simulink model "test_x_eng_nw_sim_pkt_4a_10_1"  (Simulink 7.0)
settings: Solver=ode45  StartTime=0.0  StopTime=400000  RelTol=1e-3
libraries: xbsIndex_r4 x1097, xbsReplacements_r4 x103, casper_library x28, xps_library x2, simulink x1
(part 1 of 11)
settings Model: Creator=Jason Manley  LastModifiedBy=Jason Manley
settings DebuggingCC: SaveWithParameterizedLinksMsg=none  SignalResolutionControl=TryResolveAllWithWarning  MultiTaskDSMMsg=warning  MultiTaskCondExecSysMsg=none  StrictBusMsg=None
settings RTWCC: IncludeERTFirstTime=on
settings GRTTargetCC: TargetFcnLib=ansi_tfl_tmw.mat

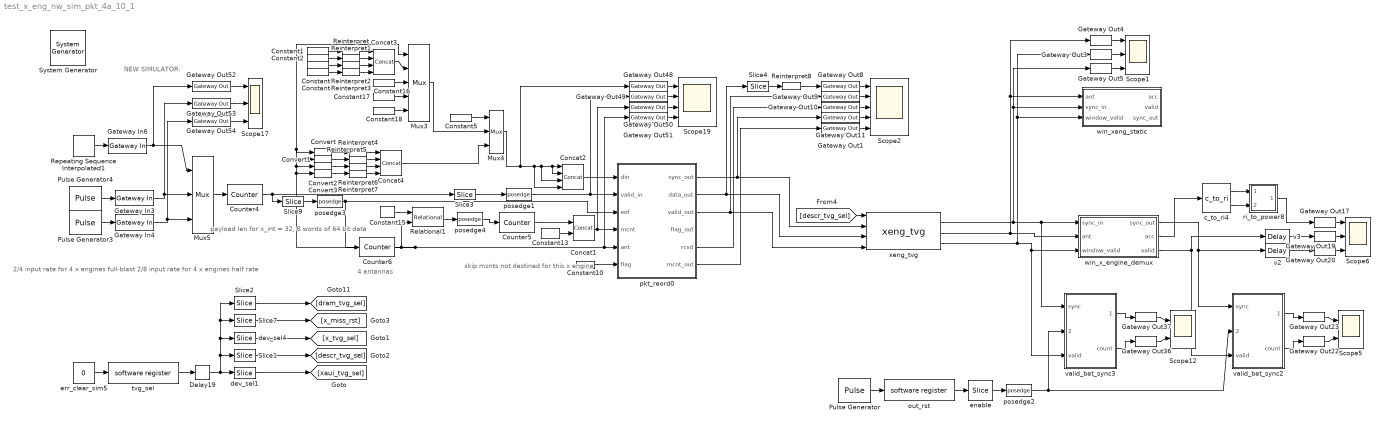
== system test_x_eng_nw_sim_pkt_4a_10_1 ==
  note: 2/4 input rate for 4 x engines full-blast
      | 2/8 input rate for 4 x engines half rate
  note: 4 antennas
  note: skip mcnts not destined
      | for this x engine
  note: payload len
      | for x_int = 32,
      | 8 words of 64 bit data
  note: NEW SIMULATOR:
  " System Generator" : xbsIndex_r4/ System Generator  Tag=genX  SystemSampleTime=-1  xilinxfamily=Virtex2  part=xc2v1000  speed=-4  package=bg575  synthesis_tool=XST  clock_wrapper=Clock Enables  directory=./netlist  testbench=off  simulink_period=1  sysclk_period=100  dcm_input_clock_period=100  incr_netlist=off  trim_vbits=Everywhere in SubSystem  dbl_ovrd=According to Block Masks  core_generation=According to Block Masks  run_coregen=off  deprecated_control=off  eval_field=0  block_type=sysgen
      settings: block_version=10.1.3
  Concat1 : xbsIndex_r4/Concat  num_inputs=2  dbl_ovrd=off  block_type=concat
      settings: block_version=10.1.3
  Concat2 : xbsIndex_r4/Concat  num_inputs=4  dbl_ovrd=off  block_type=concat
      settings: block_version=10.1.3
  Concat3 : xbsIndex_r4/Concat  num_inputs=4  dbl_ovrd=off  block_type=concat
      settings: block_version=10.1.3
  Concat4 : xbsIndex_r4/Concat  num_inputs=4  dbl_ovrd=off  block_type=concat
      settings: block_version=10.1.3
  Constant{1..4} (4 alike) : xbsIndex_r4/Constant  arith_type=Unsigned  const=0.5  n_bits=4  bin_pt=3  explicit_period=on  period=1  equ=P=C  opselect=C  inp2=PCIN>>17  opr=+  inp1=P  carry=CIN  dbl_ovrd=off  block_type=constant
  Constant10 : xbsIndex_r4/Constant  arith_type=Unsigned  const=0  n_bits=1  bin_pt=0  explicit_period=on  period=1  equ=P=C  opselect=C  inp2=PCIN>>17  opr=+  inp1=P  carry=CIN  dbl_ovrd=off  block_type=constant
  Constant13 : xbsIndex_r4/Constant  arith_type=Unsigned  const=0  n_bits=2  bin_pt=0  explicit_period=on  period=1  equ=P=C  opselect=C  inp2=PCIN>>17  opr=+  inp1=P  carry=CIN  dbl_ovrd=off  block_type=constant
  Constant15 : xbsIndex_r4/Constant  arith_type=Unsigned  const=0  n_bits=3  bin_pt=0  explicit_period=on  period=1  equ=P=C  opselect=C  inp2=PCIN>>17  opr=+  inp1=P  carry=CIN  dbl_ovrd=off  block_type=constant
  Constant16 : xbsIndex_r4/Constant  arith_type=Unsigned  const=0  n_bits=16  bin_pt=0  explicit_period=on  period=1  equ=P=C  opselect=C  inp2=PCIN>>17  opr=+  inp1=P  carry=CIN  dbl_ovrd=off  block_type=constant
  Constant17 : xbsIndex_r4/Constant  arith_type=Unsigned  const=0  n_bits=16  bin_pt=0  explicit_period=on  period=1  equ=P=C  opselect=C  inp2=PCIN>>17  opr=+  inp1=P  carry=CIN  dbl_ovrd=off  block_type=constant
  Constant18 : xbsIndex_r4/Constant  arith_type=Unsigned  const=0  n_bits=16  bin_pt=0  explicit_period=on  period=1  equ=P=C  opselect=C  inp2=PCIN>>17  opr=+  inp1=P  carry=CIN  dbl_ovrd=off  block_type=constant
  Constant5 : xbsIndex_r4/Constant  arith_type=Unsigned  const=1  n_bits=1  bin_pt=0  explicit_period=on  period=1  equ=P=C  opselect=C  inp2=PCIN>>17  opr=+  inp1=P  carry=CIN  dbl_ovrd=off  block_type=constant
  Convert{,1..3} (4 alike) : xbsIndex_r4/Convert  arith_type="Signed  (2's comp)"  n_bits=4  bin_pt=1  quantization=Truncate  overflow=Saturate  latency=0  dbl_ovrd=off  pipeline=off  block_type=convert
      settings: block_version=10.1.3
  Counter4 : xbsIndex_r4/Counter  cnt_type=Free Running  cnt_to=32  operation=Up  start_count=0  cnt_by_val=1  arith_type=Unsigned  n_bits=32  bin_pt=0  load_pin=off  rst=off  en=on  explicit_period=off  period=1  dbl_ovrd=off  use_behavioral_HDL=off  use_rpm=on  implementation=Fabric  block_type=counter
      settings: xl_area=[0, 0, 0, 0, 0, 0, 0]
  Counter5 : xbsIndex_r4/Counter  cnt_type=Free Running  cnt_to=Inf  operation=Up  start_count=0  cnt_by_val=1  arith_type=Unsigned  n_bits=48-2  bin_pt=0  load_pin=off  rst=off  en=on  explicit_period=off  period=1  dbl_ovrd=off  use_behavioral_HDL=off  use_rpm=on  implementation=Fabric  block_type=counter
      settings: xl_area=[0, 0, 0, 0, 0, 0, 0]
  Counter6 : xbsIndex_r4/Counter  cnt_type=Free Running  cnt_to=Inf  operation=Up  start_count=0  cnt_by_val=1  arith_type=Unsigned  n_bits=2  bin_pt=0  load_pin=off  rst=off  en=on  explicit_period=off  period=1  dbl_ovrd=off  use_behavioral_HDL=off  use_rpm=on  implementation=Fabric  block_type=counter
      settings: xl_area=[0, 0, 0, 0, 0, 0, 0]
  Delay19 : xbsIndex_r4/Delay  en=off  latency=2  dbl_ovrd=off  reg_retiming=off  block_type=delay
      settings: xl_area=[0, 0, 0, 0, 0, 0, 0]
  Gateway In3 : xbsIndex_r4/Gateway In  arith_type=Boolean  n_bits=8  bin_pt=6  quantization=Truncate  overflow=Wrap  period=1  dbl_ovrd=off  timing_constraint=None  locs_specified=off  LOCs={}  block_type=gatewayin
      settings: infoedit="Gateway in block.  Converts inputs of type Simulink integer, double and fixed point to  Xilinx fixed point type.<P><P>Hardware notes:  In hardware these blocks become top level input ports."  xl_area=[0, 0, 0, 0, 0, 0, 0]  block_version=10.1.3
  Gateway In4 : xbsIndex_r4/Gateway In  arith_type=Boolean  n_bits=8  bin_pt=6  quantization=Truncate  overflow=Wrap  period=1  dbl_ovrd=off  timing_constraint=None  locs_specified=off  LOCs={}  block_type=gatewayin
      settings: infoedit="Gateway in block.  Converts inputs of type Simulink integer, double and fixed point to  Xilinx fixed point type.<P><P>Hardware notes:  In hardware these blocks become top level input ports."  xl_area=[0, 0, 0, 0, 0, 0, 0]  block_version=10.1.3
  Gateway In6 : xbsIndex_r4/Gateway In  arith_type=Unsigned  n_bits=1  bin_pt=0  quantization=Truncate  overflow=Wrap  period=1  dbl_ovrd=off  timing_constraint=None  locs_specified=off  LOCs={}  block_type=gatewayin
      settings: infoedit="Gateway in block.  Converts inputs of type Simulink integer, double and fixed point to  Xilinx fixed point type.<P><P>Hardware notes:  In hardware these blocks become top level input ports."  xl_area=[0, 0, 0, 0, 0, 0, 0]  block_version=10.1.3
  Gateway Out{1,8..11,48..54} (12 alike) : xbsIndex_r4/Gateway Out  hdl_port=on  timing_constraint=None  locs_specified=off  LOCs={}  block_type=gatewayout
      settings: infoedit="Gateway out block.  Converts Xilinx fixed point inputs into ouputs of type Simulink integer, double, or fixed point.<P><P>Hardware notes:  In hardware these blocks become top level output ports or are discarded, depending on how they are configured."  xl_area=[0, 0, 0, 0, 0, 0, 0]  block_version=10.1.3
  Gateway Out{3..5,17,19..20,22..23,36..37} (10 alike) : xbsIndex_r4/Gateway Out  hdl_port=off  timing_constraint=None  locs_specified=off  LOCs={}  block_type=gatewayout
      settings: infoedit="Gateway out block.  Converts Xilinx fixed point inputs into ouputs of type Simulink integer, double, or fixed point.<P><P>Hardware notes:  In hardware these blocks become top level output ports or are discarded, depending on how they are configured."  xl_area=[0, 0, 0, 0, 0, 0, 0]  block_version=10.1.3
  Mux3 : xbsIndex_r4/Mux  inputs=4  en=off  latency=0  precision=Full  arith_type="Signed  (2's comp)"  n_bits=8  bin_pt=2  quantization=Truncate  overflow=Wrap  dbl_ovrd=off  block_type=mux
      settings: xl_area=[0, 0, 0, 0, 0, 0, 0]
  Mux4 : xbsIndex_r4/Mux  inputs=2  en=off  latency=0  precision=Full  arith_type="Signed  (2's comp)"  n_bits=8  bin_pt=2  quantization=Truncate  overflow=Wrap  dbl_ovrd=off  block_type=mux
      settings: xl_area=[0, 0, 0, 0, 0, 0, 0]
  Mux5 : xbsIndex_r4/Mux  inputs=2  en=off  latency=0  precision=Full  arith_type="Signed  (2's comp)"  n_bits=8  bin_pt=2  quantization=Truncate  overflow=Wrap  dbl_ovrd=off  block_type=mux
      settings: xl_area=[0, 0, 0, 0, 0, 0, 0]
  Pulse Generator : DiscretePulseGenerator  Period=2^15  PhaseDelay=2^14
  Pulse Generator3 : DiscretePulseGenerator  Period=4  PulseWidth=2
  Pulse Generator4 : DiscretePulseGenerator  PulseWidth=2
  Reinterpret{,1..7} (8 alike) : xbsIndex_r4/Reinterpret  force_arith_type=on  arith_type=Unsigned  force_bin_pt=on  bin_pt=0  block_type=reinterpret
      settings: infoedit="Changes signal type without altering the binary representation.   You can changed the signal between signed and unsigned, and relocate the binary point.<P><P>Hardware notes: In hardware this block costs nothing.<P><P>Example:  Suppose the input is 6 bits wide, signed, with 2 fractional bits, and the output is forced to unsigned with 0 fractional bits.  Then an input of -2.0 (1110.00 in binary 2's complement) becomes an output of 56 (111000 in binary)."  block_version=10.1.3
  Reinterpret8 : xbsIndex_r4/Reinterpret  force_arith_type=on  arith_type="Signed  (2's comp)"  force_bin_pt=on  bin_pt=3  block_type=reinterpret
      settings: infoedit="Changes signal type without altering the binary representation.   You can changed the signal between signed and unsigned, and relocate the binary point.<P><P>Hardware notes: In hardware this block costs nothing.<P><P>Example:  Suppose the input is 6 bits wide, signed, with 2 fractional bits, and the output is forced to unsigned with 0 fractional bits.  Then an input of -2.0 (1110.00 in binary 2's complement) becomes an output of 56 (111000 in binary)."  block_version=10.1.3
  Relational1 : xbsIndex_r4/Relational  mode=a=b  en=off  latency=1  dbl_ovrd=off  block_type=relational
      settings: xl_area=[0, 0, 0, 0, 0, 0, 0]  block_version=10.1.3
  Repeating Sequence Interpolated1 : simulink/Sources/Repeating Sequence Interpolated  SystemSampleTime=-1  OutValues=[0 1].'  TimeValues=[100000 300000].'  LookUpMeth=Use Input Above  tsamp=1  OutMin=[]  OutMax=[]  OutDataTypeStr=float('double')  OutputDataTypeScalingMode=Specify via dialog  OutDataType=float('double')  OutScaling=2^-10
  Scope1 : Scope  NumInputPorts=3
      settings: YMin=0~-1~0.95  YMax=1~1~1.05  SaveName=ScopeData5
  Scope12 : Scope  NumInputPorts=2
      settings: YMin=31128.7~9840  YMax=34405.3~10060  SaveName=data_into_xeng
  Scope17 : Scope  NumInputPorts=3
      settings: YMin=-1~0~0  YMax=1~1~1  SaveName=ScopeData9
  Scope19 : Scope  NumInputPorts=4
      settings: YMin=0~0~28~0  YMax=1~1~40~3  SaveName=ScopeData14
  Scope2 : Scope  NumInputPorts=5
      settings: YMin=0~0.95~0.95~-1~790  YMax=0.75~1.05~1.05~1~885
  Scope5 : Scope  NumInputPorts=2
      settings: YMin=2432~1140  YMax=2688~1150  SaveName=data_into_xeng2
  Scope6 : Scope  NumInputPorts=3
      settings: YMin=0~0~-1  YMax=1300~1~1  SaveName=ScopeData2
  Slice1 : xbsIndex_r4/Slice  nbits=2  boolean_output=off  mode=Lower Bit Location + Width  bit1=0  base1=MSB of Input  bit0=1  base0=LSB of Input  dbl_ovrd=off  block_type=slice
      settings: infoedit="Extracts a given range of bits from each input sample and presents it at the output.  The output type is ordinarily unsigned with binary point at zero, but can be Boolean when the slice is one bit wide.<P><P>Hardware notes: In hardware this block costs nothing."  block_version=10.1.3
  Slice2 : xbsIndex_r4/Slice  nbits=5  boolean_output=off  mode=Lower Bit Location + Width  bit1=0  base1=MSB of Input  bit0=9  base0=LSB of Input  dbl_ovrd=off  block_type=slice
      settings: infoedit="Extracts a given range of bits from each input sample and presents it at the output.  The output type is ordinarily unsigned with binary point at zero, but can be Boolean when the slice is one bit wide.<P><P>Hardware notes: In hardware this block costs nothing."  block_version=10.1.3
  Slice3 : xbsIndex_r4/Slice  nbits=1  boolean_output=on  mode=Lower Bit Location + Width  bit1=0  base1=MSB of Input  bit0=0  base0=LSB of Input  dbl_ovrd=off  block_type=slice
      settings: infoedit="Extracts a given range of bits from each input sample and presents it at the output.  The output type is ordinarily unsigned with binary point at zero, but can be Boolean when the slice is one bit wide.<P><P>Hardware notes: In hardware this block costs nothing."  block_version=10.1.3
  Slice4 : xbsIndex_r4/Slice  nbits=4  boolean_output=off  mode=Lower Bit Location + Width  bit1=0  base1=MSB of Input  bit0=0  base0=LSB of Input  dbl_ovrd=off  block_type=slice
      settings: infoedit="Extracts a given range of bits from each input sample and presents it at the output.  The output type is ordinarily unsigned with binary point at zero, but can be Boolean when the slice is one bit wide.<P><P>Hardware notes: In hardware this block costs nothing."  block_version=10.1.3
  Slice7 : xbsIndex_r4/Slice  nbits=1  boolean_output=on  mode=Lower Bit Location + Width  bit1=0  base1=MSB of Input  bit0=8  base0=LSB of Input  dbl_ovrd=off  block_type=slice
      settings: infoedit="Extracts a given range of bits from each input sample and presents it at the output.  The output type is ordinarily unsigned with binary point at zero, but can be Boolean when the slice is one bit wide.<P><P>Hardware notes: In hardware this block costs nothing."  block_version=10.1.3
  Slice9 : xbsIndex_r4/Slice  nbits=1  boolean_output=on  mode=Lower Bit Location + Width  bit1=0  base1=MSB of Input  bit0=4  base0=LSB of Input  dbl_ovrd=off  block_type=slice
      settings: infoedit="Extracts a given range of bits from each input sample and presents it at the output.  The output type is ordinarily unsigned with binary point at zero, but can be Boolean when the slice is one bit wide.<P><P>Hardware notes: In hardware this block costs nothing."  block_version=10.1.3
  c_to_ri4 : casper_library/Misc/c_to_ri  SystemSampleTime=-1  n_bits=16  bin_pt=6
      settings: AttributesFormatString=16_6 r/i
  dev_sel1 : xbsIndex_r4/Slice  nbits=1  boolean_output=off  mode=Lower Bit Location + Width  bit1=0  base1=MSB of Input  bit0=0  base0=LSB of Input  dbl_ovrd=off  block_type=slice
      settings: infoedit="Extracts a given range of bits from each input sample and presents it at the output.  The output type is ordinarily unsigned with binary point at zero, but can be Boolean when the slice is one bit wide.<P><P>Hardware notes: In hardware this block costs nothing."  block_version=10.1.3
  dev_sel4 : xbsIndex_r4/Slice  nbits=2  boolean_output=off  mode=Lower Bit Location + Width  bit1=0  base1=MSB of Input  bit0=3  base0=LSB of Input  dbl_ovrd=off  block_type=slice
      settings: infoedit="Extracts a given range of bits from each input sample and presents it at the output.  The output type is ordinarily unsigned with binary point at zero, but can be Boolean when the slice is one bit wide.<P><P>Hardware notes: In hardware this block costs nothing."  block_version=10.1.3
  enable : xbsIndex_r4/Slice  nbits=1  boolean_output=on  mode=Lower Bit Location + Width  bit1=0  base1=LSB of Input  bit0=0  base0=LSB of Input  dbl_ovrd=off  block_type=slice
      settings: infoedit="Extracts a given range of bits from each input sample and presents it at the output.  The output type is ordinarily unsigned with binary point at zero, but can be Boolean when the slice is one bit wide.<P><P>Hardware notes: In hardware this block costs nothing."  block_version=10.1.3
  err_clear_sim5 : Constant  Value=0  OutDataType=sfix(16)  OutScaling=2^0
  out_rst : xps_library/software register  Tag=xps:sw_reg  SystemSampleTime=-1  io_dir=From Processor  arith_type=Unsigned  bitwidth=32  bin_pt=0  sample_period=1  gw_name=test_x_eng_nw_sim_pkt_4a_10_1_out_rst_user_data_out
      link override test_x_eng_nw_sim_pkt_4a_10_1_out_rst_user_data_out: arith_type=Unsigned  n_bits=32  bin_pt=0  period=1
      link override test_x_eng_sim_packet_4a_10_1_out_rst_user_data_out: arith_type=Unsigned  n_bits=32  bin_pt=0  period=1
      link override test_x_eng_sim_pkt_4a_10_1_new_out_rst_user_data_out: arith_type=Unsigned  n_bits=32  bin_pt=0  period=1
  pkt_reord0 : Subsystem  mask{ant_bits=2, xeng_bits=2, chan_bits=10, x_int_bits=5, window_bits=3}
      mask prompts: ant_bits "Maximum Number of Antennas (2^?):"; xeng_bits "Number of Xengines in the system (2^?)"; chan_bits "Number of frequency channels in the system (2^?)"; x_int_bits "X Engine Integration Length (2^?):"; window_bits "Number of Windows to Buffer (2^?):"
      mask init:
      | sync_bits=chan_bits+x_int_bits+ant_bits-xeng_bits
      | 
      | fmtstr = sprintf('Sync period: 2^%d\nPayload Len: %i', sync_bits,2^(x_int_bits - 2));
      | set_param(gcb, 'AttributesFormatString', fmtstr);
      settings: AttributesFormatString=|
      | Sync period: 2^15
      | Payload Len: 8
  posedge{1..4} (4 alike) : casper_library/Misc/posedge  Tag=Rising Edge Detector  SystemSampleTime=-1
  ri_to_power8 : Subsystem
  tvg_sel : xps_library/software register  Tag=xps:sw_reg  SystemSampleTime=-1  io_dir=From Processor  arith_type=Unsigned  bitwidth=32  bin_pt=0  sample_period=1  gw_name=test_x_eng_nw_sim_pkt_4a_10_1_tvg_sel_user_data_out
      link override test_x_eng_nw_sim_pkt_4a_10_1_tvg_sel_user_data_out: arith_type=Unsigned  n_bits=32  bin_pt=0  period=1
      link override test_x_eng_sim_packet_4a_10_1_tvg_sel_user_data_out: arith_type=Unsigned  n_bits=32  bin_pt=0  period=1
      link override test_x_eng_sim_pkt_4a_10_1_new_tvg_sel_user_data_out: arith_type=Unsigned  n_bits=32  bin_pt=0  period=1
  v2 : xbsIndex_r4/Delay  en=off  latency=5  dbl_ovrd=off  reg_retiming=off  block_type=delay
      settings: xl_area=[0, 0, 0, 0, 0, 0, 0]
  v3 : xbsIndex_r4/Delay  en=off  latency=5  dbl_ovrd=off  reg_retiming=off  block_type=delay
      settings: xl_area=[0, 0, 0, 0, 0, 0, 0]
  valid_bet_sync2 : Subsystem
  valid_bet_sync3 : Subsystem
  win_x_engine_demux : Subsystem  AncestorBlock=casper_library/Correlator/win_x_engine_demux  mask(win_x_engine_demux){n_ants=4, n_bits=4, acc_len=32, demux_factor=8, add_latency=1, mult_latency=1, bram_latency=1, use_ded_mult=1, use_bram_delay=1}
      mask prompts: n_ants "Number of antennas"; n_bits "Bit-width of samples in"; acc_len "Accumulation length"; add_latency "Adder latency"; mult_latency "Multiplier latency"; bram_latency "BRAM latency"; use_ded_mult "Implementation: Multiplier type (0=slices 1=embedded 2=bram)"; use_bram_delay "Implementation: Delay type (0=SLR, 1=BRAM)"
      mask help: CASPER X engine with added internal valid data masking functionality and integral demux to arbitrary number of bits. Based on Aaron Parsons' and Lynn Urry's original X engine design.
      mask init:
      | xeng_delay = add_latency + mult_latency + acc_len + floor(n_ants/2 + 1) + 1;
      | bit_growth = ceil(log2(acc_len));
      | ant_bits = ceil(log2(n_ants));
      | n_bits_out = (2*n_bits + 1 + bit_growth);
      | fix_pnt_pos = (n_bits-1)*2;
      | 
      | %fprintf('Number of bits out of X engine core: %d',n_bits_out);
      | win_x_engine_demux_init(gcb, ...
      |     'n_ants', n_ants, ...
      |     'n_bits', n_bits, ...
      |     'acc_len', acc_len, ...
      |     'demux_factor', demux_factor, ...
      |     'add_latency', add_latency, ...
      |     'mult_latency', mult_latency, ...
      |     'bram_latency', bram_latency, ...
      |     'use_ded_mult', use_ded_mult, ...
      |     'use_bram_delay', use_bram_delay);
      settings: AttributesFormatString=n_ant=4, bits=4, mult=1, bram=1
  win_xeng_static : Subsystem  mask(x_engine){n_ants=4, n_bits=4, acc_len=32, add_latency=1, mult_latency=1, bram_latency=1, use_ded_mult=1, use_bram_delay=1}
      mask prompts: n_ants "Number of Antennas"; n_bits "Bit Width of Samples In"; acc_len "Accumulation Length"; add_latency "Add Latency"; mult_latency "Mult Latency"; bram_latency "BRAM Latency"; use_ded_mult "Multiplier Type (0=slices 1=embedded 2=bram)"; use_bram_delay "Delay in BRAM"
      mask init:
      | bit_growth = ceil(log2(acc_len));
      | ant_bits = ceil(log2(n_ants));
      | n_bits_out = (2*n_bits + 1 + bit_growth);
      | 
      | %win_x_engine_init(gcb, ...
      | %    'n_ants', n_ants, ...
      | %    'n_bits', n_bits, ...
      | %    'acc_len', acc_len, ...
      | %    'add_latency', add_latency, ...
      | %    'mult_latency', mult_latency, ...
      | %    'bram_latency', bram_latency, ...
      | %    'use_ded_mult', use_ded_mult, ...
      | %    'use_bram_delay', use_bram_delay);
      settings: AttributesFormatString=n_ant=4, bits=4, mult=1, bram=1
  xeng_tvg : casper_library/Correlator/xeng_tvg  SystemSampleTime=-1  ant_bits=2  x_int_bits=5  sync_period=15
      link override tv0/test_x_eng_nw_sim_pkt_4a_10_1_xeng_tvg_tv0_user_data_out: arith_type=Unsigned  n_bits=32  bin_pt=0  period=1
      link override tv1/test_x_eng_nw_sim_pkt_4a_10_1_xeng_tvg_tv1_user_data_out: arith_type=Unsigned  n_bits=32  bin_pt=0  period=1
      link override tv2/test_x_eng_nw_sim_pkt_4a_10_1_xeng_tvg_tv2_user_data_out: arith_type=Unsigned  n_bits=32  bin_pt=0  period=1
      link override tv3/test_x_eng_nw_sim_pkt_4a_10_1_xeng_tvg_tv3_user_data_out: arith_type=Unsigned  n_bits=32  bin_pt=0  period=1
      link override tv4/test_x_eng_nw_sim_pkt_4a_10_1_xeng_tvg_tv4_user_data_out: arith_type=Unsigned  n_bits=32  bin_pt=0  period=1
      link override tv5/test_x_eng_nw_sim_pkt_4a_10_1_xeng_tvg_tv5_user_data_out: arith_type=Unsigned  n_bits=32  bin_pt=0  period=1
      link override tv6/test_x_eng_nw_sim_pkt_4a_10_1_xeng_tvg_tv6_user_data_out: arith_type=Unsigned  n_bits=32  bin_pt=0  period=1
      link override tv7/test_x_eng_nw_sim_pkt_4a_10_1_xeng_tvg_tv7_user_data_out: arith_type=Unsigned  n_bits=32  bin_pt=0  period=1
  wires:
  [descr_tvg_sel] -> xeng_tvg/1
  xeng_tvg/1 -> win_xeng_static/2(sync_in), Gateway Out5/1, valid_bet_sync3/1(sync), win_x_engine_demux/1(sync_in)
  out_rst/1 -> enable/1
  Pulse Generator/1 -> out_rst/1
  enable/1 -> posedge2/1
  posedge2/1 -> valid_bet_sync3/2(rst_max), valid_bet_sync2/2(rst_max)
  Gateway Out8/1 -> Scope2/1
  Gateway Out9/1 -> Scope2/2
  Gateway Out10/1 -> Scope2/3
  Gateway Out11/1 -> Scope2/4
  pkt_reord0/1(sync_out) -> xeng_tvg/2, Gateway Out11/1
  pkt_reord0/2(data_out) -> xeng_tvg/3, Slice4/1
  err_clear_sim5/1 -> tvg_sel/1
  tvg_sel/1 -> Delay19/1
  Delay19/1 -> dev_sel1/1, Slice1/1, dev_sel4/1, Slice2/1, Slice7/1
  dev_sel1/1 -> [xaui_tvg_sel]
  Slice1/1 -> [descr_tvg_sel]
  dev_sel4/1 -> [x_tvg_sel]
  Slice7/1 -> [x_miss_rst]
  Slice2/1 -> [dram_tvg_sel]
  Gateway Out36/1 -> Scope12/2
  Gateway Out37/1 -> Scope12/1
  valid_bet_sync3/1(max_count) -> Gateway Out37/1
  valid_bet_sync3/2(count) -> Gateway Out36/1
  Constant10/1 -> pkt_reord0/6(flag)
  Gateway Out48/1 -> Scope19/1
  Gateway Out49/1 -> Scope19/2
  Gateway Out50/1 -> Scope19/3
  Gateway Out51/1 -> Scope19/4
  Constant13/1 -> Concat1/2
  Concat1/1 -> Gateway Out50/1, pkt_reord0/4(mcnt)
  Counter5/1 -> Concat1/1
  Counter6/1 -> Relational1/2, Gateway Out51/1, pkt_reord0/5(ant), Mux3/1, Convert/1, Convert1/1, Convert2/1, Convert3/1
  Concat2/1 -> pkt_reord0/1(din)
  Relational1/1 -> posedge4/1
  Constant15/1 -> Relational1/1
  Slice3/1 -> posedge1/1
  Counter4/1 -> Slice9/1, Slice3/1
  Mux4/1 -> Concat2/4, Concat2/3, Concat2/1, Concat2/2, Gateway Out48/1
  Slice9/1 -> posedge3/1
  posedge3/1 -> Counter6/1, pkt_reord0/3(eof)
  posedge4/1 -> Counter5/1
  Pulse Generator3/1 -> Gateway In4/1
  Concat3/1 -> Mux3/2
  Constant16/1 -> Mux3/3
  Constant17/1 -> Mux3/4
  Constant18/1 -> Mux3/5
  Mux3/1 -> Mux4/2
  Concat4/1 -> Mux4/3
  Constant5/1 -> Mux4/1
  Pulse Generator4/1 -> Gateway In3/1
  Mux5/1 -> Counter4/1
  Gateway In3/1 -> Gateway Out53/1, Mux5/2
  Gateway In4/1 -> Gateway Out54/1, Mux5/3
  Gateway In6/1 -> Mux5/1, Gateway Out52/1
  Repeating Sequence Interpolated1/1 -> Gateway In6/1
  Gateway Out52/1 -> Scope17/1
  Gateway Out53/1 -> Scope17/2
  Gateway Out54/1 -> Scope17/3
  xeng_tvg/3 -> valid_bet_sync3/3(valid), win_x_engine_demux/3(window_valid), win_xeng_static/3(window_valid), Gateway Out3/1
  posedge1/1 -> Gateway Out49/1, pkt_reord0/2(valid_in)
  xeng_tvg/2 -> win_xeng_static/1(ant), Gateway Out4/1, win_x_engine_demux/2(ant)
  Gateway Out3/1 -> Scope1/2
  Gateway Out4/1 -> Scope1/1
  Gateway Out5/1 -> Scope1/3
  c_to_ri4/1 -> ri_to_power8/1(In1)
  c_to_ri4/2 -> ri_to_power8/2(In2)
  Gateway Out20/1 -> Scope6/3
  Gateway Out19/1 -> Scope6/2
  Gateway Out17/1 -> Scope6/1
  ri_to_power8/1(Out1) -> Gateway Out17/1
  Gateway Out22/1 -> Scope5/2
  Gateway Out23/1 -> Scope5/1
  valid_bet_sync2/1(max_count) -> Gateway Out23/1
  valid_bet_sync2/2(count) -> Gateway Out22/1
  v2/1 -> Gateway Out20/1
  v3/1 -> Gateway Out19/1
  Constant1/1 -> Reinterpret/1
  Constant2/1 -> Reinterpret1/1
  Constant3/1 -> Reinterpret2/1
  Constant4/1 -> Reinterpret3/1
  Reinterpret/1 -> Concat3/1
  Reinterpret1/1 -> Concat3/2
  Reinterpret2/1 -> Concat3/3
  Reinterpret3/1 -> Concat3/4
  Gateway Out1/1 -> Scope2/5
  Convert/1 -> Reinterpret4/1
  Convert1/1 -> Reinterpret5/1
  Convert2/1 -> Reinterpret6/1
  Convert3/1 -> Reinterpret7/1
  Reinterpret4/1 -> Concat4/1
  Reinterpret6/1 -> Concat4/3
  Reinterpret7/1 -> Concat4/4
  Reinterpret5/1 -> Concat4/2
  Slice4/1 -> Reinterpret8/1
  Reinterpret8/1 -> Gateway Out8/1
  pkt_reord0/3(valid_out) -> xeng_tvg/4, Gateway Out9/1
  pkt_reord0/5(rcvd) -> Gateway Out10/1
  pkt_reord0/6(mcnt_out) -> Gateway Out1/1
  win_x_engine_demux/2(acc) -> c_to_ri4/1
  win_x_engine_demux/3(valid) -> v3/1, valid_bet_sync2/3(valid)
  win_x_engine_demux/1(sync_out) -> v2/1, valid_bet_sync2/1(sync)

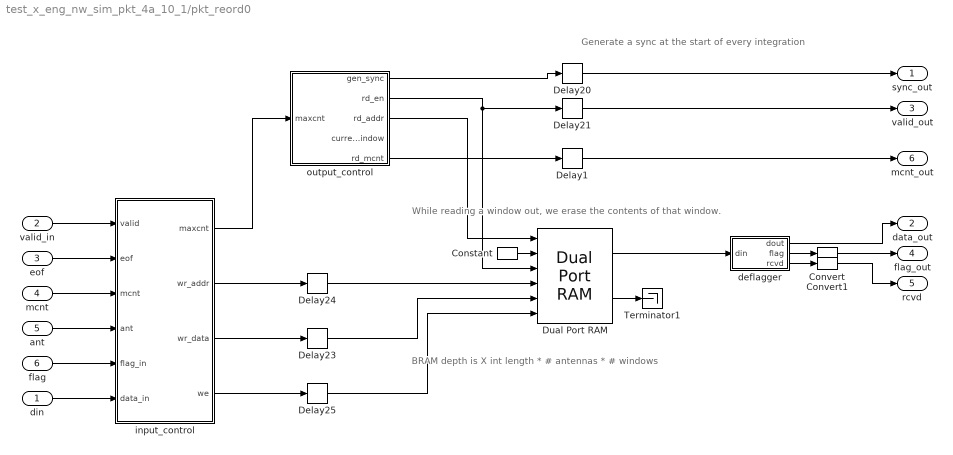
== system test_x_eng_nw_sim_pkt_4a_10_1/pkt_reord0 ==
  note: BRAM depth is
      | X int length * # antennas * # windows
  note: While reading a window out,
      | we erase the contents of that window.
  note: Generate a sync at the
      | start of every integration
  din : Inport  OutDataType=sfix(16)  OutScaling=2^0
  valid_in : Inport  Port=2  OutDataType=sfix(16)  OutScaling=2^0
  eof : Inport  Port=3  OutDataType=sfix(16)  OutScaling=2^0
  mcnt : Inport  Port=4  OutDataType=sfix(16)  OutScaling=2^0
  ant : Inport  Port=5  OutDataType=sfix(16)  OutScaling=2^0
  flag : Inport  Port=6  OutDataType=sfix(16)  OutScaling=2^0
  Constant : xbsIndex_r4/Constant  arith_type=Unsigned  const=0  n_bits=18  bin_pt=0  explicit_period=on  period=1  equ=P=C  opselect=C  inp2=PCIN>>17  opr=+  inp1=P  carry=CIN  dbl_ovrd=off  block_type=constant
  Convert : xbsIndex_r4/Convert  arith_type=Boolean  n_bits=16  bin_pt=14  quantization=Truncate  overflow=Wrap  latency=0  dbl_ovrd=off  pipeline=off  block_type=convert
      settings: block_version=10.1.3
  Convert1 : xbsIndex_r4/Convert  arith_type=Boolean  n_bits=16  bin_pt=14  quantization=Truncate  overflow=Wrap  latency=0  dbl_ovrd=off  pipeline=off  block_type=convert
      settings: block_version=10.1.3
  Delay1 : xbsIndex_r4/Delay  en=off  latency=3  dbl_ovrd=off  reg_retiming=on  block_type=delay
      settings: xl_area=[0, 0, 0, 0, 0, 0, 0]
  Delay20 : xbsIndex_r4/Delay  en=off  latency=3  dbl_ovrd=off  reg_retiming=on  block_type=delay
      settings: xl_area=[0, 0, 0, 0, 0, 0, 0]
  Delay21 : xbsIndex_r4/Delay  en=off  latency=3  dbl_ovrd=off  reg_retiming=on  block_type=delay
      settings: xl_area=[0, 0, 0, 0, 0, 0, 0]
  Delay23 : xbsIndex_r4/Delay  en=off  latency=2  dbl_ovrd=off  reg_retiming=on  block_type=delay
      settings: xl_area=[0, 0, 0, 0, 0, 0, 0]
  Delay24 : xbsIndex_r4/Delay  en=off  latency=2  dbl_ovrd=off  reg_retiming=on  block_type=delay
      settings: xl_area=[0, 0, 0, 0, 0, 0, 0]
  Delay25 : xbsIndex_r4/Delay  en=off  latency=2  dbl_ovrd=off  reg_retiming=on  block_type=delay
      settings: xl_area=[0, 0, 0, 0, 0, 0, 0]
  Dual Port RAM : xbsIndex_r4/Dual Port RAM  depth=2^x_int_bits * 2^ant_bits * 2^window_bits  initVector=1  distributed_mem=Block RAM  init_a=0  init_b=0  rst_a=off  rst_b=off  en_a=off  en_b=off  latency=3  write_mode_A=Read Before Write  write_mode_B=Read Before Write  dbl_ovrd=off  optimize=Area  use_rpm=off  block_type=dpram
      settings: xl_area=[0, 0, 0, 0, 0, 0, 0]  block_version=10.1.3
  Terminator1 : Terminator
  deflagger : Subsystem
  input_control : Subsystem
  output_control : Subsystem
  sync_out : Outport  OutDataType=sfix(16)  OutScaling=2^0
  data_out : Outport  Port=2  OutDataType=sfix(16)  OutScaling=2^0
  valid_out : Outport  Port=3  OutDataType=sfix(16)  OutScaling=2^0
  flag_out : Outport  Port=4  OutDataType=sfix(16)  OutScaling=2^0
  rcvd : Outport  Port=5  OutDataType=sfix(16)  OutScaling=2^0
  mcnt_out : Outport  Port=6  OutDataType=sfix(16)  OutScaling=2^0
  wires:
  input_control/4(we) -> Delay25/1
  input_control/2(wr_addr) -> Delay24/1
  output_control/2(rd_en) -> Dual Port RAM/3, Delay21/1
  output_control/3(rd_addr) -> Dual Port RAM/1
  Constant/1 -> Dual Port RAM/2
  deflagger/3(rcvd) -> Convert1/1
  deflagger/2(flag) -> Convert/1
  deflagger/1(dout) -> data_out/1
  Delay21/1 -> valid_out/1
  valid_in/1 -> input_control/1(valid)
  eof/1 -> input_control/2(eof)
  ant/1 -> input_control/4(ant)
  mcnt/1 -> input_control/3(mcnt)
  Delay20/1 -> sync_out/1
  Dual Port RAM/2 -> Terminator1/1
  Dual Port RAM/1 -> deflagger/1(din)
  output_control/1(gen_sync) -> Delay20/1
  input_control/3(wr_data) -> Delay23/1
  din/1 -> input_control/6(data_in)
  flag/1 -> input_control/5(flag_in)
  input_control/1(maxcnt) -> output_control/1(maxcnt)
  Delay24/1 -> Dual Port RAM/4
  Delay23/1 -> Dual Port RAM/5
  Delay25/1 -> Dual Port RAM/6
  output_control/5(rd_mcnt) -> Delay1/1
  Delay1/1 -> mcnt_out/1
  Convert/1 -> flag_out/1
  Convert1/1 -> rcvd/1

== system test_x_eng_nw_sim_pkt_4a_10_1/ri_to_power8 ==
  In1 : Inport  OutDataType=sfix(16)  OutScaling=2^0
  In2 : Inport  Orientation=down  Port=2  OutDataType=sfix(16)  OutScaling=2^0
  imag_square : xbsIndex_r4/Mult  precision=Full  arith_type="Signed  (2's comp)"  n_bits=8  bin_pt=2  quantization=Truncate  overflow=Wrap  en=off  latency=3  dbl_ovrd=off  use_behavioral_HDL=off  use_embedded=on  opt=Speed  optimum_pipeline=off  pipeline=on  use_rpm=on  placement_style=Rectangular shape  block_type=mult
      settings: infoedit=Hardware notes: To use the internal pipeline stage of the dedicated multiplier you must select 'Pipeline for maximum performance'.  xl_area=[0, 0, 0, 0, 0, 0, 0]  block_version=10.1.3
  power_adder : xbsIndex_r4/AddSub  mode=Addition  use_carryin=off  use_carryout=off  en=off  latency=2  precision=Full  arith_type=Unsigned  n_bits=8  bin_pt=2  quantization=Truncate  overflow=Wrap  dbl_ovrd=off  use_behavioral_HDL=on  pipelined=off  use_rpm=on  hw_selection=Fabric  block_type=addsub
      settings: xl_area=[0, 0, 0, 0, 0, 0, 0]  block_version=10.1.3
  real_square : xbsIndex_r4/Mult  precision=Full  arith_type="Signed  (2's comp)"  n_bits=8  bin_pt=2  quantization=Truncate  overflow=Wrap  en=off  latency=3  dbl_ovrd=off  use_behavioral_HDL=off  use_embedded=on  opt=Speed  optimum_pipeline=off  pipeline=on  use_rpm=on  placement_style=Rectangular shape  block_type=mult
      settings: infoedit=Hardware notes: To use the internal pipeline stage of the dedicated multiplier you must select 'Pipeline for maximum performance'.  xl_area=[0, 0, 0, 0, 0, 0, 0]  block_version=10.1.3
  Out1 : Outport  OutDataType=sfix(16)  OutScaling=2^0
  wires:
  power_adder/1 -> Out1/1
  In2/1 -> imag_square/2, imag_square/1
  In1/1 -> real_square/1, real_square/2
  real_square/1 -> power_adder/1
  imag_square/1 -> power_adder/2

== system test_x_eng_nw_sim_pkt_4a_10_1/valid_bet_sync2 ==
  sync : Inport  OutDataType=sfix(16)  OutScaling=2^0
  rst_max : Inport  Port=2  OutDataType=sfix(16)  OutScaling=2^0
  valid : Inport  Port=3  OutDataType=sfix(16)  OutScaling=2^0
  Delay14 : xbsIndex_r4/Delay  en=off  latency=1  dbl_ovrd=off  reg_retiming=on  block_type=delay
      settings: xl_area=[0, 0, 0, 0, 0, 0, 0]
  Register3 : xbsIndex_r4/Register  init=0  rst=on  en=on  dbl_ovrd=off  block_type=register
      settings: xl_area=[0, 0, 0, 0, 0, 0, 0]
  Relational5 : xbsIndex_r4/Relational  mode=a>=b  en=off  latency=1  dbl_ovrd=off  block_type=relational
      settings: xl_area=[0, 0, 0, 0, 0, 0, 0]  block_version=10.1.3
  valid_cntr : xbsIndex_r4/Counter  cnt_type=Count Limited  cnt_to=Inf  operation=Up  start_count=0  cnt_by_val=1  arith_type="Signed  (2's comp)"  n_bits=32  bin_pt=0  load_pin=off  rst=on  en=on  explicit_period=on  period=1  dbl_ovrd=off  use_behavioral_HDL=off  use_rpm=on  implementation=Fabric  block_type=counter
      settings: xl_area=[0, 0, 0, 0, 0, 0, 0]
  max_count : Outport  OutDataType=sfix(16)  OutScaling=2^0
  count : Outport  Port=2  OutDataType=sfix(16)  OutScaling=2^0
  wires:
  valid/1 -> valid_cntr/2
  rst_max/1 -> Register3/2
  sync/1 -> valid_cntr/1
  valid_cntr/1 -> count/1, Delay14/1, Relational5/1
  Register3/1 -> max_count/1, Relational5/2
  Relational5/1 -> Register3/3
  Delay14/1 -> Register3/1

== system test_x_eng_nw_sim_pkt_4a_10_1/valid_bet_sync3 ==
  sync : Inport  OutDataType=sfix(16)  OutScaling=2^0
  rst_max : Inport  Port=2  OutDataType=sfix(16)  OutScaling=2^0
  valid : Inport  Port=3  OutDataType=sfix(16)  OutScaling=2^0
  Delay14 : xbsIndex_r4/Delay  en=off  latency=1  dbl_ovrd=off  reg_retiming=on  block_type=delay
      settings: xl_area=[0, 0, 0, 0, 0, 0, 0]
  Register3 : xbsIndex_r4/Register  init=0  rst=on  en=on  dbl_ovrd=off  block_type=register
      settings: xl_area=[0, 0, 0, 0, 0, 0, 0]
  Relational5 : xbsIndex_r4/Relational  mode=a>=b  en=off  latency=1  dbl_ovrd=off  block_type=relational
      settings: xl_area=[0, 0, 0, 0, 0, 0, 0]  block_version=10.1.3
  valid_cntr : xbsIndex_r4/Counter  cnt_type=Count Limited  cnt_to=Inf  operation=Up  start_count=0  cnt_by_val=1  arith_type="Signed  (2's comp)"  n_bits=32  bin_pt=0  load_pin=off  rst=on  en=on  explicit_period=on  period=1  dbl_ovrd=off  use_behavioral_HDL=off  use_rpm=on  implementation=Fabric  block_type=counter
      settings: xl_area=[0, 0, 0, 0, 0, 0, 0]
  max_count : Outport  OutDataType=sfix(16)  OutScaling=2^0
  count : Outport  Port=2  OutDataType=sfix(16)  OutScaling=2^0
  wires:
  Delay14/1 -> Register3/1
  Relational5/1 -> Register3/3
  Register3/1 -> Relational5/2, max_count/1
  valid_cntr/1 -> Relational5/1, Delay14/1, count/1
  sync/1 -> valid_cntr/1
  rst_max/1 -> Register3/2
  valid/1 -> valid_cntr/2

== system test_x_eng_nw_sim_pkt_4a_10_1/win_x_engine_demux ==
  sync_in : Inport
  ant : Inport  Port=2
  window_valid : Inport  Port=3
  Constant : xbsIndex_r4/Constant  arith_type=Unsigned  const=0  n_bits=112  bin_pt=14  explicit_period=off  period=1  equ=P=C  opselect=C  inp2=PCIN>>17  opr=+  inp1=P  carry=CIN  dbl_ovrd=off  block_type=constant
  Constant1 : xbsIndex_r4/Constant  arith_type=Boolean  const=0  n_bits=1  bin_pt=14  explicit_period=off  period=1  equ=P=C  opselect=C  inp2=PCIN>>17  opr=+  inp1=P  carry=CIN  dbl_ovrd=off  block_type=constant
  Logical : xbsIndex_r4/Logical  logical_function=AND  inputs=2  en=off  latency=0  precision=Full  arith_type=Unsigned  n_bits=16  bin_pt=0  align_bp=on  dbl_ovrd=off  block_type=logical
  Term1 : Terminator
  Term2 : Terminator
  Term3 : Terminator
  auto_tap : casper_library/Correlator/auto_tap  SystemSampleTime=-1  use_ded_mult=1
      settings: AttributesFormatString=mult=1
  baseline_tap1 : casper_library/Correlator/baseline_tap  SystemSampleTime=-1  ant_sep=1  use_ded_mult=1  use_bram_delay=1
      settings: AttributesFormatString=ant_sep=1, mult=1, bram=1
  baseline_tap2 : Subsystem  AncestorBlock=casper_library/Correlator/baseline_tap  mask(baseline_tap){ant_sep=2, use_ded_mult=1, use_bram_delay=1}
      mask prompts: ant_sep "Antenna Seperation"; use_ded_mult "Multiplier Type (0=slices 1=embedded 2=bram)"; use_bram_delay "Delay in BRAM"
      mask init:
      | baseline_tap_init(gcb, ...
      |     'ant_sep', ant_sep, ...
      |     'use_ded_mult', use_ded_mult, ...
      |     'use_bram_delay', use_bram_delay);
      settings: AttributesFormatString=ant_sep=2, mult=1, bram=1
  window_delay : casper_library/Delays/window_delay  SystemSampleTime=-1  delay=38
  x_cast : casper_library/Correlator/x_cast  SystemSampleTime=-1  n_bits_in=14  n_bits_out=16  fix_pnt_pos=6
  xeng_conj_fix : Subsystem  AncestorBlock=casper_library/Correlator/xeng_conj_fix  mask(xeng_conj_fix){n_ants=4, n_bits_in=8, demux_factor=8}
      mask prompts: n_ants "Number of Antennas"; n_bits_in "Input Bitwidth (complex, bit width per component)"; demux_factor "Demux factor"
      mask help:
      | This block corrects the "lower triangle" of the X engine's output so that products are conjugated according to the astronomy convention of
      | lower_antenna_index * conj(higher_antenna_index).
      |
      | It expects demuxed input. Ie the ACC line contains a single complex number per clock.
      mask init:
      | xeng_conj_fix_init(gcb, 'n_ants', n_ants,...
      |     'n_bits_in',n_bits_in,...
      |     'demux_factor',demux_factor);
      | 
      | fmtstr = sprintf('num_ants=%d',n_ants);
      | set_param(gcb, 'AttributesFormatString', fmtstr);
      settings: AttributesFormatString=num_ants=4
  xeng_mask_demux : casper_library/Correlator/xeng_mask_demux  SystemSampleTime=-1  num_ants=4  n_bits_in=128  demux_factor=8
      settings: AttributesFormatString=num_ants=4
  sync_out : Outport
  acc : Outport  Port=2
  valid : Outport  Port=3
  wires:
  ant/1 -> auto_tap/1, auto_tap/2
  Constant/1 -> auto_tap/4
  Constant1/1 -> auto_tap/5
  sync_in/1 -> auto_tap/6
  window_valid/1 -> window_delay/1
  window_delay/1 -> Logical/2
  Logical/1 -> xeng_mask_demux/2
  x_cast/1 -> xeng_mask_demux/1
  xeng_mask_demux/1 -> xeng_conj_fix/1(acc)
  xeng_mask_demux/2 -> xeng_conj_fix/2(valid)
  xeng_mask_demux/3 -> xeng_conj_fix/3(sync)
  xeng_conj_fix/3(sync_out) -> sync_out/1
  xeng_conj_fix/1(acc_out) -> acc/1
  xeng_conj_fix/2(valid_out) -> valid/1
  auto_tap/1 -> baseline_tap1/1
  auto_tap/2 -> baseline_tap1/2
  auto_tap/3 -> baseline_tap1/3
  auto_tap/4 -> baseline_tap1/4
  auto_tap/5 -> baseline_tap1/5
  auto_tap/6 -> baseline_tap1/6
  auto_tap/7 -> baseline_tap1/7
  baseline_tap1/1 -> baseline_tap2/1(a_del)
  baseline_tap1/2 -> baseline_tap2/2(a_ndel)
  baseline_tap1/3 -> baseline_tap2/3(a_end)
  baseline_tap1/4 -> baseline_tap2/4(acc_in)
  baseline_tap1/5 -> baseline_tap2/5(valid_in)
  baseline_tap1/6 -> baseline_tap2/6(rst)
  baseline_tap1/7 -> baseline_tap2/7(sync1)
  baseline_tap2/1(a_del_out) -> auto_tap/3
  baseline_tap2/2(a_ndel_out) -> Term1/1
  baseline_tap2/3(a_end_out) -> Term2/1
  baseline_tap2/4(acc_out) -> x_cast/1
  baseline_tap2/5(valid_out) -> Logical/1
  baseline_tap2/6(rst_out) -> Term3/1
  baseline_tap2/7(sync_out) -> xeng_mask_demux/3

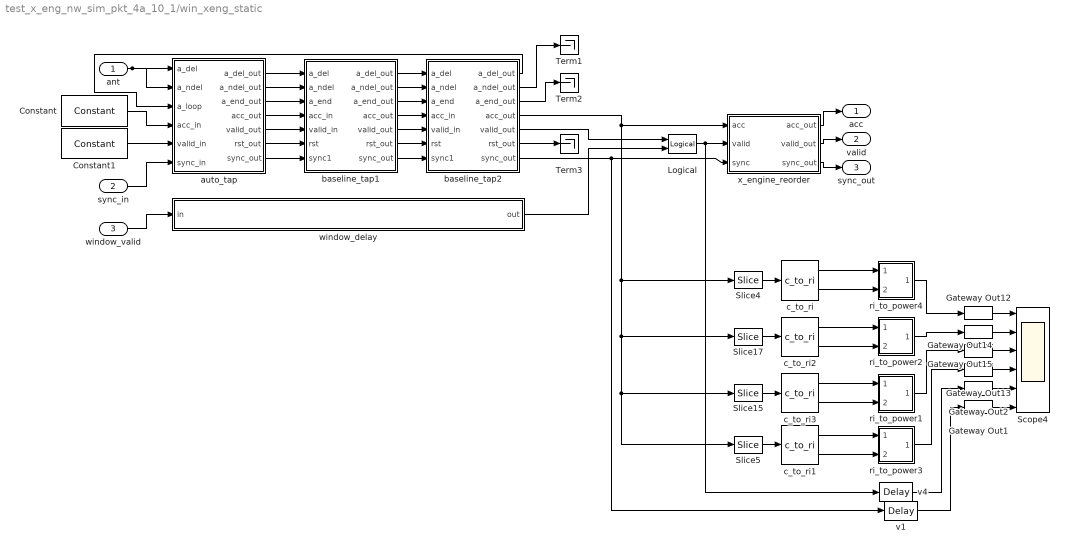
== system test_x_eng_nw_sim_pkt_4a_10_1/win_xeng_static ==
  ant : Inport  OutDataType=sfix(16)  OutScaling=2^0
  sync_in : Inport  Port=2  OutDataType=sfix(16)  OutScaling=2^0
  window_valid : Inport  Port=3  OutDataType=sfix(16)  OutScaling=2^0
  Constant : xbsIndex_r4/Constant  arith_type=Unsigned  const=0  n_bits=8 * n_bits_out  bin_pt=0  explicit_period=on  period=1  equ=P=C  opselect=C  inp2=PCIN>>17  opr=+  inp1=P  carry=CIN  dbl_ovrd=off  block_type=constant
  Constant1 : xbsIndex_r4/Constant  arith_type=Boolean  const=0  n_bits=1  bin_pt=0  explicit_period=on  period=1  equ=P=C  opselect=C  inp2=PCIN>>17  opr=+  inp1=P  carry=CIN  dbl_ovrd=off  block_type=constant
  Gateway Out{1..2,12..15} (6 alike) : xbsIndex_r4/Gateway Out  hdl_port=off  timing_constraint=None  locs_specified=off  LOCs={}  block_type=gatewayout
      settings: infoedit="Gateway out block.  Converts Xilinx fixed point inputs into ouputs of type Simulink integer, double, or fixed point.<P><P>Hardware notes:  In hardware these blocks become top level output ports or are discarded, depending on how they are configured."  xl_area=[0, 0, 0, 0, 0, 0, 0]  block_version=10.1.3
  Logical : xbsIndex_r4/Logical  logical_function=AND  inputs=2  en=off  latency=0  precision=Full  arith_type=Unsigned  n_bits=8  bin_pt=2  align_bp=on  dbl_ovrd=off  block_type=logical
      settings: xl_area=[0, 0, 0, 0, 0, 0, 0]
  Scope4 : Scope  NumInputPorts=6
      settings: YMin=0~0~0~0~0~-1  YMax=1300~1300~1300~1300~1~1  SaveName=ScopeData2
  Slice15 : xbsIndex_r4/Slice  nbits=112/4  boolean_output=off  mode=Lower Bit Location + Width  bit1=0  base1=MSB of Input  bit0=112/4  base0=LSB of Input  dbl_ovrd=off  block_type=slice
      settings: infoedit="Extracts a given range of bits from each input sample and presents it at the output.  The output type is ordinarily unsigned with binary point at zero, but can be Boolean when the slice is one bit wide.<P><P>Hardware notes: In hardware this block costs nothing."  block_version=10.1.3
  Slice17 : xbsIndex_r4/Slice  nbits=112/4  boolean_output=off  mode=Lower Bit Location + Width  bit1=0  base1=MSB of Input  bit0=112/4*2  base0=LSB of Input  dbl_ovrd=off  block_type=slice
      settings: infoedit="Extracts a given range of bits from each input sample and presents it at the output.  The output type is ordinarily unsigned with binary point at zero, but can be Boolean when the slice is one bit wide.<P><P>Hardware notes: In hardware this block costs nothing."  block_version=10.1.3
  Slice4 : xbsIndex_r4/Slice  nbits=112/4  boolean_output=off  mode=Lower Bit Location + Width  bit1=0  base1=MSB of Input  bit0=112/4*3  base0=LSB of Input  dbl_ovrd=off  block_type=slice
      settings: infoedit="Extracts a given range of bits from each input sample and presents it at the output.  The output type is ordinarily unsigned with binary point at zero, but can be Boolean when the slice is one bit wide.<P><P>Hardware notes: In hardware this block costs nothing."  block_version=10.1.3
  Slice5 : xbsIndex_r4/Slice  nbits=112/4  boolean_output=off  mode=Lower Bit Location + Width  bit1=0  base1=MSB of Input  bit0=0  base0=LSB of Input  dbl_ovrd=off  block_type=slice
      settings: infoedit="Extracts a given range of bits from each input sample and presents it at the output.  The output type is ordinarily unsigned with binary point at zero, but can be Boolean when the slice is one bit wide.<P><P>Hardware notes: In hardware this block costs nothing."  block_version=10.1.3
  Term1 : Terminator
  Term2 : Terminator
  Term3 : Terminator
  auto_tap : Subsystem  mask(auto_tap){use_ded_mult=1}
      mask prompts: use_ded_mult "Use Dedicated Multipliers"
      mask init:
      | auto_tap_init(gcb, ...
      |     'use_ded_mult', use_ded_mult);
      settings: AttributesFormatString=mult=1
  baseline_tap1 : Subsystem  mask(baseline_tap){ant_sep=1, use_ded_mult=1, use_bram_delay=1}
      mask prompts: ant_sep "Antenna Seperation"; use_ded_mult "Multiplier Type (0=slices 1=embedded 2=bram)"; use_bram_delay "Delay in BRAM"
      mask init:
      | %baseline_tap_init(gcb, ...
      | %    'ant_sep', ant_sep, ...
      | %    'use_ded_mult', use_ded_mult, ...
      | %    'use_bram_delay', use_bram_delay);
      settings: AttributesFormatString=ant_sep=1, mult=1, bram=1
  baseline_tap2 : Subsystem  mask(baseline_tap){ant_sep=2, use_ded_mult=1, use_bram_delay=1}
      mask prompts: ant_sep "Antenna Seperation"; use_ded_mult "Multiplier Type (0=slices 1=embedded 2=bram)"; use_bram_delay "Delay in BRAM"
      mask init:
      | %baseline_tap_init(gcb, ...
      | %    'ant_sep', ant_sep, ...
      | %    'use_ded_mult', use_ded_mult, ...
      | %    'use_bram_delay', use_bram_delay);
      settings: AttributesFormatString=ant_sep=1, mult=1, bram=1
  c_to_ri{,1..3} (4 alike) : casper_library/Misc/c_to_ri  SystemSampleTime=-1  n_bits=14  bin_pt=6
      settings: AttributesFormatString=14_6 r/i
  ri_to_power1 : Subsystem
  ri_to_power2 : Subsystem
  ri_to_power3 : Subsystem
  ri_to_power4 : Subsystem
  v1 : xbsIndex_r4/Delay  en=off  latency=5  dbl_ovrd=off  reg_retiming=off  block_type=delay
      settings: xl_area=[0, 0, 0, 0, 0, 0, 0]
  v4 : xbsIndex_r4/Delay  en=off  latency=5  dbl_ovrd=off  reg_retiming=off  block_type=delay
      settings: xl_area=[0, 0, 0, 0, 0, 0, 0]
  window_delay : Subsystem  mask{delay=add_latency + mult_latency + acc_len + floor(n_ants/2 + 1) + 1}
      mask prompts: delay "desired delay (>2)"
      mask Display: fprintf('Z^-%d', delay)
  x_engine_reorder : Subsystem  mask{num_ants=n_ants}
      mask prompts: num_ants "Number of Antennas"
      mask init:
      | num_taps = floor(num_ants/2) + 1;
      | num_validins = num_ants*num_taps;
      | 
      | addr_offset = floor(num_ants/2) * num_taps - sum(1:num_taps-1) - 1;
      | if (mod(num_ants, 2) == 0)
      |     addr_offset = addr_offset - floor(num_ants/2);
      | end
      | 
      | num_elements = nchoosek(num_ants, 2) + num_ants;
      | elements_bits = floor(log2(num_elements)) + 1;
      | 
      | fmtstr = sprintf('num_ants=%d',num_ants);
      | set_param(gcb, 'AttributesFormatString', fmtstr);
      settings: AttributesFormatString=num_ants=4
  acc : Outport  OutDataType=sfix(16)  OutScaling=2^0
  valid : Outport  Port=2  OutDataType=sfix(16)  OutScaling=2^0
  sync_out : Outport  Port=3  OutDataType=sfix(16)  OutScaling=2^0
  wires:
  Slice4/1 -> c_to_ri/1
  Slice17/1 -> c_to_ri2/1
  Slice15/1 -> c_to_ri3/1
  Slice5/1 -> c_to_ri1/1
  c_to_ri/1 -> ri_to_power4/1(In1)
  c_to_ri/2 -> ri_to_power4/2(In2)
  c_to_ri2/1 -> ri_to_power2/1(In1)
  c_to_ri2/2 -> ri_to_power2/2(In2)
  c_to_ri3/1 -> ri_to_power1/1(In1)
  c_to_ri3/2 -> ri_to_power1/2(In2)
  c_to_ri1/1 -> ri_to_power3/1(In1)
  c_to_ri1/2 -> ri_to_power3/2(In2)
  Gateway Out15/1 -> Scope4/3
  Gateway Out14/1 -> Scope4/2
  Gateway Out12/1 -> Scope4/1
  Gateway Out13/1 -> Scope4/4
  ri_to_power4/1(Out1) -> Gateway Out12/1
  ri_to_power2/1(Out1) -> Gateway Out14/1
  ri_to_power1/1(Out1) -> Gateway Out15/1
  ri_to_power3/1(Out1) -> Gateway Out13/1
  Gateway Out2/1 -> Scope4/5
  Gateway Out1/1 -> Scope4/6
  v1/1 -> Gateway Out1/1
  v4/1 -> Gateway Out2/1
  ant/1 -> auto_tap/1(a_del), auto_tap/2(a_ndel)
  x_engine_reorder/1(acc_out) -> acc/1
  x_engine_reorder/2(valid_out) -> valid/1
  x_engine_reorder/3(sync_out) -> sync_out/1
  Logical/1 -> x_engine_reorder/2(valid), v4/1
  Constant/1 -> auto_tap/4(acc_in)
  Constant1/1 -> auto_tap/5(valid_in)
  sync_in/1 -> auto_tap/6(sync_in)
  window_valid/1 -> window_delay/1(in)
  window_delay/1(out) -> Logical/2
  auto_tap/1(a_del_out) -> baseline_tap1/1(a_del)
  auto_tap/2(a_ndel_out) -> baseline_tap1/2(a_ndel)
  auto_tap/3(a_end_out) -> baseline_tap1/3(a_end)
  auto_tap/4(acc_out) -> baseline_tap1/4(acc_in)
  auto_tap/5(valid_out) -> baseline_tap1/5(valid_in)
  auto_tap/6(rst_out) -> baseline_tap1/6(rst)
  auto_tap/7(sync_out) -> baseline_tap1/7(sync1)
  baseline_tap1/1(a_del_out) -> baseline_tap2/1(a_del)
  baseline_tap1/2(a_ndel_out) -> baseline_tap2/2(a_ndel)
  baseline_tap1/3(a_end_out) -> baseline_tap2/3(a_end)
  baseline_tap1/4(acc_out) -> baseline_tap2/4(acc_in)
  baseline_tap1/5(valid_out) -> baseline_tap2/5(valid_in)
  baseline_tap1/6(rst_out) -> baseline_tap2/6(rst)
  baseline_tap1/7(sync_out) -> baseline_tap2/7(sync1)
  baseline_tap2/1(a_del_out) -> auto_tap/3(a_loop)
  baseline_tap2/2(a_ndel_out) -> Term1/1
  baseline_tap2/3(a_end_out) -> Term2/1
  baseline_tap2/4(acc_out) -> x_engine_reorder/1(acc), Slice4/1, Slice17/1, Slice5/1, Slice15/1
  baseline_tap2/5(valid_out) -> Logical/1
  baseline_tap2/6(rst_out) -> Term3/1
  baseline_tap2/7(sync_out) -> x_engine_reorder/3(sync), v1/1

== system test_x_eng_nw_sim_pkt_4a_10_1/pkt_reord0/deflagger ==
  din : Inport  OutDataType=sfix(16)  OutScaling=2^0
  Slice1 : xbsIndex_r4/Slice  nbits=16  boolean_output=off  mode=Lower Bit Location + Width  bit1=0  base1=MSB of Input  bit0=0  base0=LSB of Input  dbl_ovrd=off  block_type=slice
      settings: infoedit="Extracts a given range of bits from each input sample and presents it at the output.  The output type is ordinarily unsigned with binary point at zero, but can be Boolean when the slice is one bit wide.<P><P>Hardware notes: In hardware this block costs nothing."  block_version=10.1.3
  Slice2 : xbsIndex_r4/Slice  nbits=1  boolean_output=off  mode=Upper Bit Location + Width  bit1=-1  base1=MSB of Input  bit0=0  base0=LSB of Input  dbl_ovrd=off  block_type=slice
      settings: infoedit="Extracts a given range of bits from each input sample and presents it at the output.  The output type is ordinarily unsigned with binary point at zero, but can be Boolean when the slice is one bit wide.<P><P>Hardware notes: In hardware this block costs nothing."  block_version=10.1.3
  Slice3 : xbsIndex_r4/Slice  nbits=1  boolean_output=off  mode=Upper Bit Location + Width  bit1=0  base1=MSB of Input  bit0=0  base0=LSB of Input  dbl_ovrd=off  block_type=slice
      settings: infoedit="Extracts a given range of bits from each input sample and presents it at the output.  The output type is ordinarily unsigned with binary point at zero, but can be Boolean when the slice is one bit wide.<P><P>Hardware notes: In hardware this block costs nothing."  block_version=10.1.3
  dout : Outport  OutDataType=sfix(16)  OutScaling=2^0
  flag : Outport  Port=2  OutDataType=sfix(16)  OutScaling=2^0
  rcvd : Outport  Port=3  OutDataType=sfix(16)  OutScaling=2^0
  wires:
  Slice1/1 -> dout/1
  Slice3/1 -> rcvd/1
  Slice2/1 -> flag/1
  din/1 -> Slice3/1, Slice2/1, Slice1/1
